simulink model "gm_fft_overlap_tomori"  (R2023b)
settings: Solver=VariableStepAuto  StartTime=0.0  StopTime=inf  RelTol=1e-3
InitFcn:
  | fftparrallelout
  | load('dataram.mat')
  | s= fi(exp(-1j*2*pi.*(0:63)/64),1,16,15);
  | fixed_point = fixdt(1,27,20);
  | fixed_pointu = fixdt(0,29,20);
  | fixed = fixdt(1,22,15);
  | const = fixdt(1,18,17);
  | addConst = fixdt(1,18,16);
  | f =10.4e6;
  | f1=45e6;
  | alpha1 =5;
  | beta1 = 0.00001 ;
  | beta2 = 0.99999 ;
  | beta3 = 23;
undefined symbols (not defined in the file or in its folder): j
libraries: dspxfrm3 x11, commrflib2 x4
(part 1 of 10)
settings Model: Creator=ehsan  LastModifiedBy=mori
settings OptimizationCC: BlockReduction=off  ConditionallyExecuteInputs=off  ReuseModelBlockBuffer=off
settings DebuggingCC: InheritedTsInSrcMsg=none

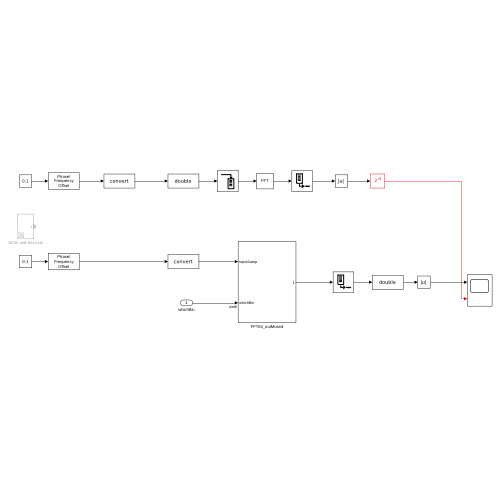
[thumbnail: Simulink's stored preview of the top-level diagram]
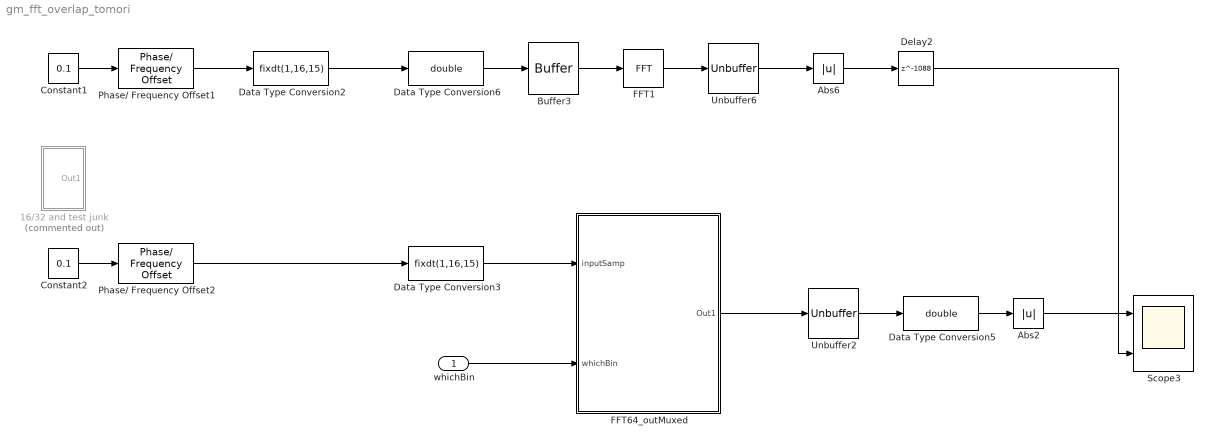
== system gm_fft_overlap_tomori ==
  whichBin : Inport
  16/32 and test junk : Subsystem  Commented=on
  Abs2 : Abs  SaturateOnIntegerOverflow=off
  Abs6 : Abs  SaturateOnIntegerOverflow=off
  Buffer3 : Buffer  V=63  OutputFrames=off
  Constant1 : Constant  Value=0.1  SampleTime=2e-8
  Constant2 : Constant  Value=0.1  SampleTime=2e-8
  Data Type Conversion2 : DataTypeConversion  OutDataTypeStr=fixdt(1,16,15)  SaturateOnIntegerOverflow=off  RndMeth=Floor
  Data Type Conversion3 : DataTypeConversion  OutDataTypeStr=fixdt(1,16,15)  SaturateOnIntegerOverflow=off  RndMeth=Floor
  Data Type Conversion5 : DataTypeConversion  OutDataTypeStr=double  SaturateOnIntegerOverflow=off  RndMeth=Floor
  Data Type Conversion6 : DataTypeConversion  OutDataTypeStr=double  SaturateOnIntegerOverflow=off  RndMeth=Floor
  Delay2 : Delay  DelayLength=1088
  FFT1 : dspxfrm3/FFT  FFTImplementation=Auto  CompMethod=Table lookup  TableOpt=NEW  TableOptActive=Speed  BitRevOrder=off  Normalize=off  InheritFFTLength=on  FFTLength=64  WrapInput=on  roundingMode=Floor  overflowMode=off  firstCoeffDataTypeStr=Inherit: Same word length as input  firstCoeffLastDataTypeStr=Inherit: Same word length as input  outputMin=[]  outputMax=[]
  FFT64_outMuxed : Subsystem
  Phase/ Frequency Offset1 : commrflib2/Phase// Frequency Offset  phaseOffset=0  freqPort=off  freqOffset=1e6
  Phase/ Frequency Offset2 : commrflib2/Phase// Frequency Offset  phaseOffset=0  freqPort=off  freqOffset=1e6
  Scope3 : Scope  NumInputPorts=2
  Unbuffer2 : Unbuffer
  Unbuffer6 : Unbuffer
  wires:
  whichBin/1 -> FFT64_outMuxed/2(whichBin)
  FFT64_outMuxed/1(Out1) -> Unbuffer2/1
  Data Type Conversion3/1 -> FFT64_outMuxed/1(inputSamp)
  Data Type Conversion2/1 -> Data Type Conversion6/1
  Phase/ Frequency Offset1/1 -> Data Type Conversion2/1
  Constant1/1 -> Phase/ Frequency Offset1/1
  Delay2/1 -> Scope3/2
  Abs6/1 -> Delay2/1
  Unbuffer6/1 -> Abs6/1
  FFT1/1 -> Unbuffer6/1
  Buffer3/1 -> FFT1/1
  Abs2/1 -> Scope3/1
  Data Type Conversion5/1 -> Abs2/1
  Unbuffer2/1 -> Data Type Conversion5/1
  Constant2/1 -> Phase/ Frequency Offset2/1
  Phase/ Frequency Offset2/1 -> Data Type Conversion3/1
  Data Type Conversion6/1 -> Buffer3/1

== system gm_fft_overlap_tomori/16//32 and test junk ==
  16 : Subsystem  Commented=on
  16pointfftchan1 : Subsystem  Commented=on
  32 : Subsystem  Commented=on
  Discrete FIR Filter : DiscreteFir  Commented=on  Coefficients=ones(1, 32)
  Real-Imag to Complex : RealImagToComplex  Commented=on
  Sine Wave2 : Sin  Commented=on  Frequency=2*pi*1e6  SampleTime=2e-8
  Sine Wave3 : Sin  Commented=on  Amplitude=.99  Frequency=2*pi*1e6  Phase=pi/2  SampleTime=2e-8
  Out1 : Outport
  wires:
  Real-Imag to Complex/1 -> Out1/1
  Sine Wave3/1 -> Real-Imag to Complex/1
  Sine Wave2/1 -> Real-Imag to Complex/2

== system gm_fft_overlap_tomori/FFT64_outMuxed ==
  inputSamp : Inport
  whichBin : Inport  Port=2  OutDataTypeStr=uint8
  64pointFFTchan : Subsystem
  Multiport Switch1 : MultiPortSwitch  DataPortOrder=Zero-based contiguous  Inputs=64  zeroidx=on  SaturateOnIntegerOverflow=off  InputSameDT=off
  Out1 : Outport
  wires:
  64pointFFTchan/64(Out64) -> Multiport Switch1/65
  64pointFFTchan/63(Out63) -> Multiport Switch1/64
  64pointFFTchan/1(Out1) -> Multiport Switch1/2
  64pointFFTchan/62(Out62) -> Multiport Switch1/63
  64pointFFTchan/2(Out2) -> Multiport Switch1/3
  64pointFFTchan/61(Out61) -> Multiport Switch1/62
  64pointFFTchan/3(Out3) -> Multiport Switch1/4
  64pointFFTchan/60(Out60) -> Multiport Switch1/61
  64pointFFTchan/4(Out4) -> Multiport Switch1/5
  64pointFFTchan/59(Out59) -> Multiport Switch1/60
  64pointFFTchan/5(Out5) -> Multiport Switch1/6
  64pointFFTchan/58(Out58) -> Multiport Switch1/59
  64pointFFTchan/6(Out6) -> Multiport Switch1/7
  64pointFFTchan/57(Out57) -> Multiport Switch1/58
  64pointFFTchan/7(Out7) -> Multiport Switch1/8
  64pointFFTchan/56(Out56) -> Multiport Switch1/57
  64pointFFTchan/8(Out8) -> Multiport Switch1/9
  64pointFFTchan/55(Out55) -> Multiport Switch1/56
  64pointFFTchan/9(Out9) -> Multiport Switch1/10
  64pointFFTchan/54(Out54) -> Multiport Switch1/55
  64pointFFTchan/10(Out10) -> Multiport Switch1/11
  64pointFFTchan/53(Out53) -> Multiport Switch1/54
  64pointFFTchan/11(Out11) -> Multiport Switch1/12
  64pointFFTchan/52(Out52) -> Multiport Switch1/53
  64pointFFTchan/12(Out12) -> Multiport Switch1/13
  64pointFFTchan/51(Out51) -> Multiport Switch1/52
  64pointFFTchan/13(Out13) -> Multiport Switch1/14
  64pointFFTchan/50(Out50) -> Multiport Switch1/51
  64pointFFTchan/14(Out14) -> Multiport Switch1/15
  64pointFFTchan/49(Out49) -> Multiport Switch1/50
  64pointFFTchan/15(Out15) -> Multiport Switch1/16
  64pointFFTchan/48(Out48) -> Multiport Switch1/49
  64pointFFTchan/16(Out16) -> Multiport Switch1/17
  64pointFFTchan/47(Out47) -> Multiport Switch1/48
  64pointFFTchan/17(Out17) -> Multiport Switch1/18
  64pointFFTchan/46(Out46) -> Multiport Switch1/47
  64pointFFTchan/18(Out18) -> Multiport Switch1/19
  64pointFFTchan/45(Out45) -> Multiport Switch1/46
  64pointFFTchan/19(Out19) -> Multiport Switch1/20
  64pointFFTchan/44(Out44) -> Multiport Switch1/45
  64pointFFTchan/20(Out20) -> Multiport Switch1/21
  64pointFFTchan/43(Out43) -> Multiport Switch1/44
  64pointFFTchan/21(Out21) -> Multiport Switch1/22
  64pointFFTchan/42(Out42) -> Multiport Switch1/43
  64pointFFTchan/22(Out22) -> Multiport Switch1/23
  64pointFFTchan/41(Out41) -> Multiport Switch1/42
  64pointFFTchan/23(Out23) -> Multiport Switch1/24
  64pointFFTchan/40(Out40) -> Multiport Switch1/41
  64pointFFTchan/24(Out24) -> Multiport Switch1/25
  64pointFFTchan/39(Out39) -> Multiport Switch1/40
  64pointFFTchan/25(Out25) -> Multiport Switch1/26
  64pointFFTchan/38(Out38) -> Multiport Switch1/39
  64pointFFTchan/26(Out26) -> Multiport Switch1/27
  64pointFFTchan/37(Out37) -> Multiport Switch1/38
  64pointFFTchan/27(Out27) -> Multiport Switch1/28
  64pointFFTchan/36(Out36) -> Multiport Switch1/37
  64pointFFTchan/28(Out28) -> Multiport Switch1/29
  64pointFFTchan/35(Out35) -> Multiport Switch1/36
  64pointFFTchan/29(Out29) -> Multiport Switch1/30
  64pointFFTchan/34(Out34) -> Multiport Switch1/35
  64pointFFTchan/30(Out30) -> Multiport Switch1/31
  64pointFFTchan/33(Out33) -> Multiport Switch1/34
  64pointFFTchan/31(Out31) -> Multiport Switch1/32
  64pointFFTchan/32(Out32) -> Multiport Switch1/33
  whichBin/1 -> Multiport Switch1/1
  inputSamp/1 -> 64pointFFTchan/1(inputSamp)
  Multiport Switch1/1 -> Out1/1

== system gm_fft_overlap_tomori/16//32 and test junk/16 ==
  Abs4 : Abs  SaturateOnIntegerOverflow=off
  Abs5 : Abs  SaturateOnIntegerOverflow=off
  Buffer2 : Buffer  N=16  V=15  OutputFrames=off
  Constant1 : Constant  Value=0.9  SampleTime=2e-8
  Data Type Conversion10 : DataTypeConversion  SaturateOnIntegerOverflow=off  RndMeth=Floor
  Data Type Conversion12 : DataTypeConversion  OutDataTypeStr=double  SaturateOnIntegerOverflow=off  RndMeth=Floor
  Data Type Conversion8 : DataTypeConversion  OutDataTypeStr=fixdt(1,16,15)  SaturateOnIntegerOverflow=off  RndMeth=Floor
  Data Type Conversion9 : DataTypeConversion  OutDataTypeStr=fixdt(1,16,15)  SaturateOnIntegerOverflow=off  RndMeth=Floor
  Delay{34..48} (15 alike) : Delay  DelayLength=1
  Delay49 : Delay  DelayLength=416-272
  FFT16 : Subsystem
  FFT4 : dspxfrm3/FFT  FFTImplementation=Auto  CompMethod=Table lookup  TableOpt=NEW  TableOptActive=Speed  BitRevOrder=off  Normalize=off  InheritFFTLength=on  FFTLength=64  WrapInput=on  roundingMode=Floor  overflowMode=off  firstCoeffDataTypeStr=Inherit: Same word length as input  firstCoeffLastDataTypeStr=Inherit: Same word length as input  outputMin=[]  outputMax=[]
  Mux1 : Mux  Inputs=16
  Phase/ Frequency Offset1 : commrflib2/Phase// Frequency Offset  phaseOffset=pi/2*180/pi  freqPort=off  freqOffset=1e6
  Scope8 : Scope  NumInputPorts=2
  Unbuffer4 : Unbuffer
  Unbuffer5 : Unbuffer
  wires:
  FFT16/14(x13) -> Mux1/14
  Delay37/1 -> Delay38/1, FFT16/5(In5)
  FFT16/12(x11) -> Mux1/12
  Abs4/1 -> Delay49/1
  FFT16/6(x5) -> Mux1/6
  FFT16/16(x15) -> Mux1/16
  FFT16/4(x3) -> Mux1/4
  Buffer2/1 -> FFT4/1
  Delay45/1 -> Delay46/1, FFT16/13(In13)
  FFT16/3(x2) -> Mux1/3
  Delay48/1 -> FFT16/16(In16)
  Delay42/1 -> Delay43/1, FFT16/10(In10)
  Delay36/1 -> Delay37/1, FFT16/4(In4)
  FFT16/1(x0) -> Mux1/1
  FFT16/7(x6) -> Mux1/7
  Delay43/1 -> Delay44/1, FFT16/11(In11)
  FFT16/15(x14) -> Mux1/15
  Data Type Conversion8/1 -> Delay34/1, FFT16/1(In1)
  Delay41/1 -> Delay42/1, FFT16/9(In9)
  Delay34/1 -> Delay35/1, FFT16/2(In2)
  FFT16/9(x8) -> Mux1/9
  FFT16/13(x12) -> Mux1/13
  Delay40/1 -> Delay41/1, FFT16/8(In8)
  Delay49/1 -> Scope8/1
  Unbuffer4/1 -> Abs4/1
  FFT16/2(x1) -> Mux1/2
  FFT16/5(x4) -> Mux1/5
  Data Type Conversion10/1 -> Buffer2/1
  Phase/ Frequency Offset1/1 -> Data Type Conversion8/1, Data Type Conversion9/1
  Mux1/1 -> Unbuffer5/1
  Delay46/1 -> Delay47/1, FFT16/14(In14)
  Delay39/1 -> Delay40/1, FFT16/7(In7)
  Data Type Conversion9/1 -> Data Type Conversion10/1
  Delay47/1 -> Delay48/1, FFT16/15(In15)
  Constant1/1 -> Phase/ Frequency Offset1/1
  FFT16/8(x7) -> Mux1/8
  FFT16/10(x9) -> Mux1/10
  FFT16/11(x10) -> Mux1/11
  Unbuffer5/1 -> Data Type Conversion12/1
  Delay44/1 -> Delay45/1, FFT16/12(In12)
  Data Type Conversion12/1 -> Abs5/1
  Delay35/1 -> Delay36/1, FFT16/3(In3)
  Delay38/1 -> Delay39/1, FFT16/6(In6)
  Abs5/1 -> Scope8/2
  FFT4/1 -> Unbuffer4/1

== system gm_fft_overlap_tomori/16//32 and test junk/16pointfftchan1 ==
  Input : Inport
      settings: SignalType=complex
  Delay{10..24} (15 alike) : Delay  DelayLength=1
  fft_res : Subsystem
  Out1 : Outport
  wires:
  Delay24/1 -> fft_res/16(In16)
  Delay11/1 -> Delay12/1, fft_res/3(In3)
  Delay15/1 -> fft_res/7(In7), Delay16/1
  Delay13/1 -> fft_res/5(In5), Delay14/1
  Delay20/1 -> fft_res/12(In12), Delay21/1
  Delay14/1 -> fft_res/6(In6), Delay15/1
  Delay22/1 -> fft_res/14(In14), Delay23/1
  Delay19/1 -> fft_res/11(In11), Delay20/1
  Delay23/1 -> fft_res/15(In15), Delay24/1
  Input/1 -> fft_res/1(In1), Delay10/1
  Delay12/1 -> fft_res/4(In4), Delay13/1
  Delay17/1 -> Delay18/1, fft_res/9(In9)
  Delay10/1 -> Delay11/1, fft_res/2(In2)
  Delay18/1 -> fft_res/10(In10), Delay19/1
  fft_res/1(Out1) -> Out1/1
  Delay16/1 -> fft_res/8(In8), Delay17/1
  Delay21/1 -> fft_res/13(In13), Delay22/1

== system gm_fft_overlap_tomori/16//32 and test junk/32 ==
  In1 : Inport
  Abs1 : Abs  SaturateOnIntegerOverflow=off
  Abs3 : Abs  SaturateOnIntegerOverflow=off
  Buffer : Buffer  Commented=on  V=63  OutputFrames=off
  Buffer1 : Buffer  N=32  V=31  OutputFrames=off
  Constant : Constant  Value=0.1  SampleTime=2e-8
  Data Type Conversion : DataTypeConversion  Commented=on  OutDataTypeStr=fixdt(1,16,15)  SaturateOnIntegerOverflow=off  RndMeth=Floor
  Data Type Conversion1 : DataTypeConversion  OutDataTypeStr=fixdt(1,16,15)  SaturateOnIntegerOverflow=off  RndMeth=Floor
  Data Type Conversion4 : DataTypeConversion  OutDataTypeStr=double  SaturateOnIntegerOverflow=off  RndMeth=Floor
  Delay1 : Delay  DelayLength=416
  Delay{3..33} (31 alike) : Delay  DelayLength=1
  FFT : dspxfrm3/FFT  Commented=on  FFTImplementation=Auto  CompMethod=Table lookup  TableOpt=NEW  TableOptActive=Speed  BitRevOrder=off  Normalize=off  InheritFFTLength=on  FFTLength=64  WrapInput=on  roundingMode=Floor  overflowMode=off  firstCoeffDataTypeStr=Inherit: Same word length as input  firstCoeffLastDataTypeStr=Inherit: Same word length as input  outputMin=[]  outputMax=[]
  FFT2 : dspxfrm3/FFT  FFTImplementation=Auto  CompMethod=Table lookup  TableOpt=NEW  TableOptActive=Speed  BitRevOrder=off  Normalize=off  InheritFFTLength=on  FFTLength=64  WrapInput=on  roundingMode=Floor  overflowMode=off  firstCoeffDataTypeStr=Inherit: Same word length as input  firstCoeffLastDataTypeStr=Inherit: Same word length as input  outputMin=[]  outputMax=[]
  FFT32 : Subsystem
  Mux : Mux  Inputs=32
  Phase/ Frequency Offset : commrflib2/Phase// Frequency Offset  phaseOffset=0  freqPort=off  freqOffset=1e6
  Scope : Scope  Commented=on
  Scope1 : Scope  NumInputPorts=2
  Scope10 : Scope  NumInputPorts=2
  Scope2 : Scope
  Sine Wave : Sin  Commented=on  Frequency=2*pi*12.5e6  SampleTime=0
  Spectrum Analyzer : SpectrumAnalyzer  Commented=on
  Unbuffer1 : Unbuffer
  Unbuffer3 : Unbuffer
  wires:
  FFT32/6(x5) -> Mux/6
  In1/1 -> Buffer1/1
  FFT32/17(x16) -> Mux/17
  Buffer/1 -> FFT/1
  FFT32/9(x8) -> Mux/9
  Delay25/1 -> FFT32/25(In25), Delay26/1
  Delay14/1 -> Delay15/1, FFT32/6(In6)
  Delay26/1 -> FFT32/26(In26), Delay27/1
  FFT32/21(x20) -> Mux/21
  Data Type Conversion4/1 -> Scope10/2, Abs1/1
  Delay13/1 -> Delay14/1, FFT32/5(In5)
  FFT32/31(x30) -> Mux/31
  Delay22/1 -> Delay23/1, FFT32/14(In14)
  Delay9/1 -> FFT32/24(In24), Delay25/1
  FFT32/2(x1) -> Mux/2
  Unbuffer3/1 -> Scope10/1, Abs3/1
  FFT/1 -> Spectrum Analyzer/1
  FFT32/28(x27) -> Mux/28
  Data Type Conversion/1 -> Scope/1, Buffer/1
  FFT32/1(x0) -> Mux/1
  Delay3/1 -> FFT32/17(In19), Delay33/1
  Delay24/1 -> Delay3/1, FFT32/16(In17)
  Delay32/1 -> FFT32/32(In32)
  Delay18/1 -> Delay19/1, FFT32/10(In10)
  Phase/ Frequency Offset/1 -> Data Type Conversion1/1
  FFT32/18(x17) -> Mux/18
  Delay29/1 -> FFT32/29(In29), Delay30/1
  Abs1/1 -> Scope2/1, Scope1/1
  Delay6/1 -> FFT32/21(In21), Delay7/1
  Mux/1 -> Unbuffer1/1
  FFT32/23(x22) -> Mux/23
  Delay30/1 -> FFT32/30(In30), Delay31/1
  FFT32/20(x19) -> Mux/20
  Delay1/1 -> Scope1/2
  Delay5/1 -> FFT32/20(In20), Delay6/1
  Delay17/1 -> Delay18/1, FFT32/9(In9)
  Delay27/1 -> FFT32/27(In27), Delay28/1
  FFT32/8(x7) -> Mux/8
  Sine Wave/1 -> Data Type Conversion/1
  Delay23/1 -> Delay24/1, FFT32/15(In15)
  Delay20/1 -> Delay21/1, FFT32/12(In12)
  FFT32/10(x9) -> Mux/10
  Delay12/1 -> Delay13/1, FFT32/4(In4)
  Unbuffer1/1 -> Data Type Conversion4/1
  FFT32/29(x28) -> Mux/29
  Delay33/1 -> FFT32/18(In16), Delay4/1
  Delay19/1 -> Delay20/1, FFT32/11(In11)
  FFT32/27(x26) -> Mux/27
  FFT32/25(x24) -> Mux/25
  Data Type Conversion1/1 -> Delay10/1, FFT32/1(In1)
  Delay4/1 -> FFT32/19(In18), Delay5/1
  FFT32/30(x29) -> Mux/30
  Constant/1 -> Phase/ Frequency Offset/1
  Delay15/1 -> Delay16/1, FFT32/7(In7)
  Delay11/1 -> Delay12/1, FFT32/3(In3)
  FFT2/1 -> Unbuffer3/1
  FFT32/19(x18) -> Mux/19
  FFT32/11(x10) -> Mux/11
  FFT32/13(x12) -> Mux/13
  Delay8/1 -> FFT32/23(In23), Delay9/1
  Delay7/1 -> FFT32/22(In22), Delay8/1
  Delay10/1 -> Delay11/1, FFT32/2(In2)
  Delay31/1 -> FFT32/31(In31), Delay32/1
  Delay16/1 -> Delay17/1, FFT32/8(In8)
  FFT32/3(x2) -> Mux/3
  FFT32/24(x23) -> Mux/24
  Delay28/1 -> FFT32/28(In28), Delay29/1
  FFT32/5(x4) -> Mux/5
  FFT32/14(x13) -> Mux/14
  Delay21/1 -> Delay22/1, FFT32/13(In13)
  FFT32/32(x31) -> Mux/32
  FFT32/15(x14) -> Mux/15
  FFT32/12(x11) -> Mux/12
  FFT32/4(x3) -> Mux/4
  FFT32/16(x15) -> Mux/16
  Buffer1/1 -> FFT2/1
  FFT32/22(x21) -> Mux/22
  Abs3/1 -> Delay1/1
  FFT32/26(x25) -> Mux/26
  FFT32/7(x6) -> Mux/7

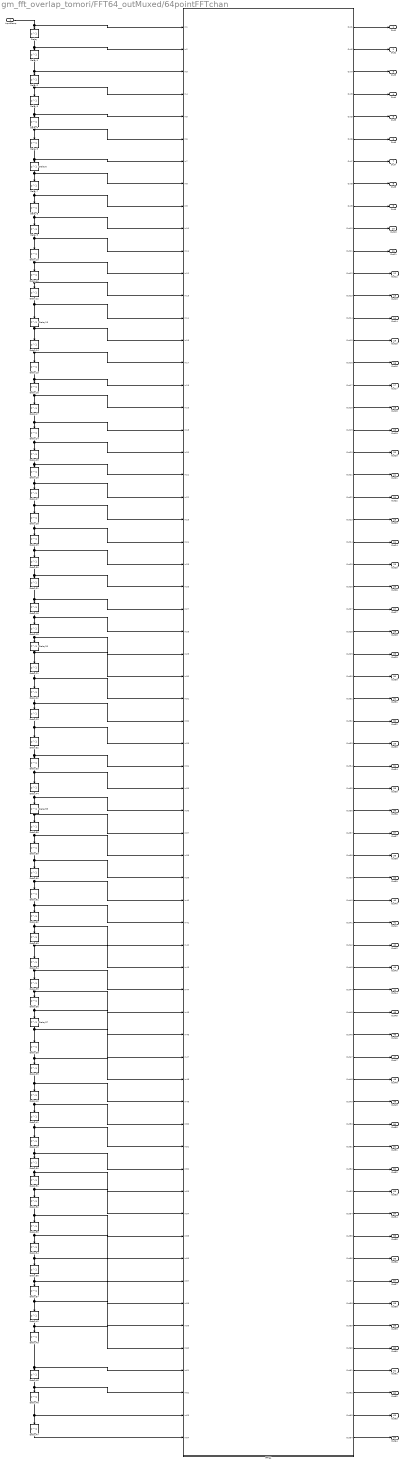
== system gm_fft_overlap_tomori/FFT64_outMuxed/64pointFFTchan ==
  inputSamp : Inport  OutDataTypeStr=fixdt(1,16, 15)
  Delay{,1..47,49..63} (63 alike) : Delay  DelayLength=1
  FFT64 : Subsystem
  Out1 : Outport  VectorParamsAs1DForOutWhenUnconnected=off
  Out2 : Outport  Port=2  VectorParamsAs1DForOutWhenUnconnected=off
  Out3 : Outport  Port=3  VectorParamsAs1DForOutWhenUnconnected=off
  Out4 : Outport  Port=4  VectorParamsAs1DForOutWhenUnconnected=off
  Out5 : Outport  Port=5  VectorParamsAs1DForOutWhenUnconnected=off
  Out6 : Outport  Port=6  VectorParamsAs1DForOutWhenUnconnected=off
  Out7 : Outport  Port=7  VectorParamsAs1DForOutWhenUnconnected=off
  Out8 : Outport  Port=8  VectorParamsAs1DForOutWhenUnconnected=off
  Out9 : Outport  Port=9  VectorParamsAs1DForOutWhenUnconnected=off
  Out10 : Outport  Port=10  VectorParamsAs1DForOutWhenUnconnected=off
  Out11 : Outport  Port=11  VectorParamsAs1DForOutWhenUnconnected=off
  Out12 : Outport  Port=12  VectorParamsAs1DForOutWhenUnconnected=off
  Out13 : Outport  Port=13  VectorParamsAs1DForOutWhenUnconnected=off
  Out14 : Outport  Port=14  VectorParamsAs1DForOutWhenUnconnected=off
  Out15 : Outport  Port=15  VectorParamsAs1DForOutWhenUnconnected=off
  Out16 : Outport  Port=16  VectorParamsAs1DForOutWhenUnconnected=off
  Out17 : Outport  Port=17  VectorParamsAs1DForOutWhenUnconnected=off
  Out18 : Outport  Port=18  VectorParamsAs1DForOutWhenUnconnected=off
  Out19 : Outport  Port=19  VectorParamsAs1DForOutWhenUnconnected=off
  Out20 : Outport  Port=20  VectorParamsAs1DForOutWhenUnconnected=off
  Out21 : Outport  Port=21  VectorParamsAs1DForOutWhenUnconnected=off
  Out22 : Outport  Port=22  VectorParamsAs1DForOutWhenUnconnected=off
  Out23 : Outport  Port=23  VectorParamsAs1DForOutWhenUnconnected=off
  Out24 : Outport  Port=24  VectorParamsAs1DForOutWhenUnconnected=off
  Out25 : Outport  Port=25  VectorParamsAs1DForOutWhenUnconnected=off
  Out26 : Outport  Port=26  VectorParamsAs1DForOutWhenUnconnected=off
  Out27 : Outport  Port=27  VectorParamsAs1DForOutWhenUnconnected=off
  Out28 : Outport  Port=28  VectorParamsAs1DForOutWhenUnconnected=off
  Out29 : Outport  Port=29  VectorParamsAs1DForOutWhenUnconnected=off
  Out30 : Outport  Port=30  VectorParamsAs1DForOutWhenUnconnected=off
  Out31 : Outport  Port=31  VectorParamsAs1DForOutWhenUnconnected=off
  Out32 : Outport  Port=32  VectorParamsAs1DForOutWhenUnconnected=off
  Out33 : Outport  Port=33  VectorParamsAs1DForOutWhenUnconnected=off
  Out34 : Outport  Port=34  VectorParamsAs1DForOutWhenUnconnected=off
  Out35 : Outport  Port=35  VectorParamsAs1DForOutWhenUnconnected=off
  Out36 : Outport  Port=36  VectorParamsAs1DForOutWhenUnconnected=off
  Out37 : Outport  Port=37  VectorParamsAs1DForOutWhenUnconnected=off
  Out38 : Outport  Port=38  VectorParamsAs1DForOutWhenUnconnected=off
  Out39 : Outport  Port=39  VectorParamsAs1DForOutWhenUnconnected=off
  Out40 : Outport  Port=40  VectorParamsAs1DForOutWhenUnconnected=off
  Out41 : Outport  Port=41  VectorParamsAs1DForOutWhenUnconnected=off
  Out42 : Outport  Port=42  VectorParamsAs1DForOutWhenUnconnected=off
  Out43 : Outport  Port=43  VectorParamsAs1DForOutWhenUnconnected=off
  Out44 : Outport  Port=44  VectorParamsAs1DForOutWhenUnconnected=off
  Out45 : Outport  Port=45  VectorParamsAs1DForOutWhenUnconnected=off
  Out46 : Outport  Port=46  VectorParamsAs1DForOutWhenUnconnected=off
  Out47 : Outport  Port=47  VectorParamsAs1DForOutWhenUnconnected=off
  Out48 : Outport  Port=48  VectorParamsAs1DForOutWhenUnconnected=off
  Out49 : Outport  Port=49  VectorParamsAs1DForOutWhenUnconnected=off
  Out50 : Outport  Port=50  VectorParamsAs1DForOutWhenUnconnected=off
  Out51 : Outport  Port=51  VectorParamsAs1DForOutWhenUnconnected=off
  Out52 : Outport  Port=52  VectorParamsAs1DForOutWhenUnconnected=off
  Out53 : Outport  Port=53  VectorParamsAs1DForOutWhenUnconnected=off
  Out54 : Outport  Port=54  VectorParamsAs1DForOutWhenUnconnected=off
  Out55 : Outport  Port=55  VectorParamsAs1DForOutWhenUnconnected=off
  Out56 : Outport  Port=56  VectorParamsAs1DForOutWhenUnconnected=off
  Out57 : Outport  Port=57  VectorParamsAs1DForOutWhenUnconnected=off
  Out58 : Outport  Port=58  VectorParamsAs1DForOutWhenUnconnected=off
  Out59 : Outport  Port=59  VectorParamsAs1DForOutWhenUnconnected=off
  Out60 : Outport  Port=60  VectorParamsAs1DForOutWhenUnconnected=off
  Out61 : Outport  Port=61  VectorParamsAs1DForOutWhenUnconnected=off
  Out62 : Outport  Port=62  VectorParamsAs1DForOutWhenUnconnected=off
  Out63 : Outport  Port=63  VectorParamsAs1DForOutWhenUnconnected=off
  Out64 : Outport  Port=64  VectorParamsAs1DForOutWhenUnconnected=off
  wires:
  FFT64/64(Out64) -> Out64/1
  FFT64/63(Out63) -> Out63/1
  FFT64/62(Out62) -> Out62/1
  FFT64/61(Out61) -> Out61/1
  FFT64/60(Out60) -> Out60/1
  FFT64/59(Out59) -> Out59/1
  FFT64/58(Out58) -> Out58/1
  FFT64/57(Out57) -> Out57/1
  FFT64/56(Out56) -> Out56/1
  FFT64/55(Out55) -> Out55/1
  FFT64/54(Out54) -> Out54/1
  FFT64/53(Out53) -> Out53/1
  FFT64/52(Out52) -> Out52/1
  FFT64/51(Out51) -> Out51/1
  FFT64/50(Out50) -> Out50/1
  FFT64/49(Out49) -> Out49/1
  FFT64/48(Out48) -> Out48/1
  FFT64/47(Out47) -> Out47/1
  FFT64/46(Out46) -> Out46/1
  FFT64/45(Out45) -> Out45/1
  FFT64/44(Out44) -> Out44/1
  FFT64/43(Out43) -> Out43/1
  FFT64/42(Out42) -> Out42/1
  FFT64/41(Out41) -> Out41/1
  FFT64/40(Out40) -> Out40/1
  FFT64/39(Out39) -> Out39/1
  FFT64/38(Out38) -> Out38/1
  FFT64/37(Out37) -> Out37/1
  FFT64/36(Out36) -> Out36/1
  FFT64/35(Out35) -> Out35/1
  FFT64/34(Out34) -> Out34/1
  FFT64/33(Out33) -> Out33/1
  FFT64/32(Out32) -> Out32/1
  FFT64/31(Out31) -> Out31/1
  FFT64/30(Out30) -> Out30/1
  FFT64/29(Out29) -> Out29/1
  FFT64/28(Out28) -> Out28/1
  FFT64/27(Out27) -> Out27/1
  FFT64/26(Out26) -> Out26/1
  FFT64/25(Out25) -> Out25/1
  FFT64/24(Out24) -> Out24/1
  FFT64/23(Out23) -> Out23/1
  FFT64/22(Out22) -> Out22/1
  FFT64/21(Out21) -> Out21/1
  FFT64/20(Out20) -> Out20/1
  FFT64/19(Out19) -> Out19/1
  FFT64/18(Out18) -> Out18/1
  FFT64/17(Out17) -> Out17/1
  FFT64/16(Out16) -> Out16/1
  FFT64/15(Out15) -> Out15/1
  FFT64/14(Out14) -> Out14/1
  FFT64/13(Out13) -> Out13/1
  FFT64/12(Out12) -> Out12/1
  FFT64/11(Out11) -> Out11/1
  FFT64/10(Out10) -> Out10/1
  FFT64/9(Out9) -> Out9/1
  FFT64/8(Out8) -> Out8/1
  FFT64/7(Out7) -> Out7/1
  FFT64/6(Out6) -> Out6/1
  FFT64/5(Out5) -> Out5/1
  FFT64/4(Out3) -> Out4/1
  FFT64/3(Out4) -> Out3/1
  FFT64/2(Out2) -> Out2/1
  FFT64/1(Out1) -> Out1/1
  Delay47/1 -> FFT64/64(In64)
  Delay23/1 -> Delay32/1, FFT64/33(In33)
  Delay32/1 -> Delay33/1, FFT64/34(In34)
  Delay44/1 -> Delay55/1, FFT64/36(In36)
  Delay33/1 -> Delay44/1, FFT64/35(In35)
  Delay58/1 -> Delay59/1, FFT64/38(In38)
  Delay59/1 -> Delay60/1, FFT64/39(In39)
  Delay60/1 -> Delay61/1, FFT64/40(In40)
  Delay55/1 -> Delay58/1, FFT64/37(In37)
  Delay35/1 -> Delay36/1, FFT64/45(In45)
  Delay38/1 -> Delay39/1, FFT64/48(In48)
  Delay37/1 -> Delay38/1, FFT64/47(In47)
  Delay36/1 -> Delay37/1, FFT64/46(In46)
  Delay63/1 -> Delay34/1, FFT64/43(In43)
  Delay34/1 -> Delay35/1, FFT64/44(In44)
  Delay62/1 -> Delay63/1, FFT64/42(In42)
  Delay61/1 -> Delay62/1, FFT64/41(In41)
  Delay42/1 -> Delay43/1, FFT64/60(In60)
  Delay56/1 -> Delay57/1, FFT64/58(In58)
  Delay45/1 -> Delay46/1, FFT64/62(In62)
  Delay50/1 -> Delay51/1, FFT64/53(In53)
  Delay49/1 -> Delay50/1, FFT64/52(In52)
  Delay51/1 -> Delay52/1, FFT64/54(In54)
  Delay41/1 -> Delay49/1, FFT64/51(In51)
  Delay46/1 -> Delay47/1, FFT64/63(In63)
  Delay53/1 -> Delay54/1, FFT64/56(In56)
  Delay57/1 -> Delay42/1, FFT64/59(In59)
  Delay52/1 -> Delay53/1, FFT64/55(In55)
  Delay43/1 -> Delay45/1, FFT64/61(In61)
  Delay40/1 -> Delay41/1, FFT64/50(In50)
  Delay54/1 -> Delay56/1, FFT64/57(In57)
  Delay39/1 -> Delay40/1, FFT64/49(In49)
  Delay15/1 -> Delay16/1, FFT64/17(In19)
  Delay29/1 -> Delay30/1, FFT64/25(In25)
  Delay16/1 -> Delay17/1, FFT64/18(In16)
  Delay19/1 -> Delay20/1, FFT64/29(In29)
  Delay27/1 -> Delay28/1, FFT64/23(In23)
  Delay31/1 -> Delay18/1, FFT64/27(In27)
  Delay28/1 -> Delay29/1, FFT64/24(In24)
  Delay21/1 -> Delay22/1, FFT64/31(In31)
  Delay17/1 -> Delay24/1, FFT64/19(In18)
  Delay26/1 -> Delay27/1, FFT64/22(In22)
  Delay24/1 -> Delay25/1, FFT64/20(In20)
  Delay22/1 -> Delay23/1, FFT64/32(In32)
  Delay25/1 -> Delay26/1, FFT64/21(In21)
  Delay20/1 -> Delay21/1, FFT64/30(In30)
  Delay30/1 -> Delay31/1, FFT64/26(In26)
  Delay18/1 -> Delay19/1, FFT64/28(In28)
  Delay7/1 -> Delay8/1, FFT64/9(In9)
  Delay8/1 -> Delay9/1, FFT64/10(In10)
  Delay10/1 -> Delay11/1, FFT64/12(In12)
  Delay9/1 -> Delay10/1, FFT64/11(In11)
  Delay12/1 -> Delay13/1, FFT64/14(In14)
  Delay13/1 -> Delay14/1, FFT64/15(In15)
  Delay14/1 -> Delay15/1, FFT64/16(In17)
  Delay11/1 -> Delay12/1, FFT64/13(In13)
  Delay3/1 -> Delay4/1, FFT64/5(In5)
  Delay6/1 -> Delay7/1, FFT64/8(In8)
  Delay5/1 -> Delay6/1, FFT64/7(In7)
  Delay4/1 -> Delay5/1, FFT64/6(In6)
  Delay1/1 -> Delay2/1, FFT64/3(In3)
  Delay2/1 -> Delay3/1, FFT64/4(In4)
  Delay/1 -> Delay1/1, FFT64/2(In2)
  inputSamp/1 -> Delay/1, FFT64/1(In1)

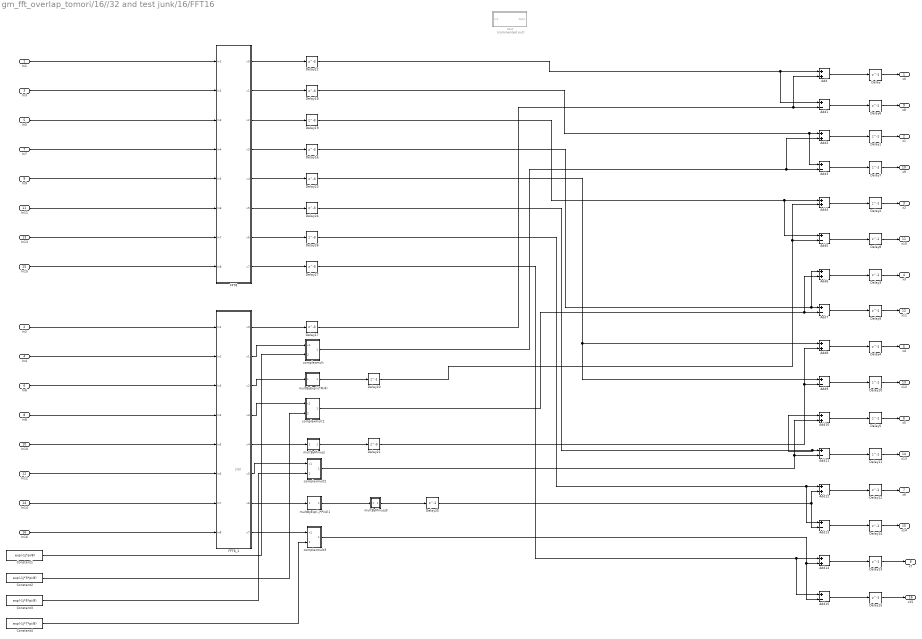
== system gm_fft_overlap_tomori/16//32 and test junk/16/FFT16 ==
  note: s(5)
  In1 : Inport
  In2 : Inport  Port=2
  In3 : Inport  Port=3
  In4 : Inport  Port=4
  In5 : Inport  Port=5
  In6 : Inport  Port=6
  In7 : Inport  Port=7
  In8 : Inport  Port=8
  In9 : Inport  Port=9
  In10 : Inport  Port=10
  In11 : Inport  Port=11
  In12 : Inport  Port=12
  In13 : Inport  Port=13
  In14 : Inport  Port=14
  In15 : Inport  Port=15
  In16 : Inport  Port=16
  Add{,2,4,6,8,10,12,14} (8 alike) : Sum  OutDataTypeStr=fixed
  Add{1,3,5,7,9,11,13,15} (8 alike) : Sum  Inputs=+-  OutDataTypeStr=fixed
  Constant1 : Constant  Value=exp(-1j*pi/8)  OutDataTypeStr=fixed  SampleTime=-1
  Constant2 : Constant  Value=exp(-1j*3*pi/8)  OutDataTypeStr=fixed  SampleTime=-1
  Constant3 : Constant  Value=exp(-1j*5*pi/8)  OutDataTypeStr=fixed  SampleTime=-1
  Constant4 : Constant  Value=exp(-1j*7*pi/8)  OutDataTypeStr=fixed  SampleTime=-1
  Delay{,1..15,20,25} (18 alike) : Delay  DelayLength=1
  Delay{16..19,21..24,26..27} (10 alike) : Delay  DelayLength=3
  FFT8 : Subsystem
  FFT8_1 : Subsystem
  complexmult : Subsystem
  complexmult1 : Subsystem
  complexmult2 : Subsystem
  complexmult3 : Subsystem
  multByExp(-j*Pi/4) : Subsystem
  multByExp(-j*Pi/4)1 : Subsystem
  multByMinusJ : Subsystem
  multByMinusJ3 : Subsystem
  test : Subsystem  Commented=on
  x0 : Outport
  x1 : Outport  Port=2
  x2 : Outport  Port=3
  x3 : Outport  Port=4
  x4 : Outport  Port=5
  x5 : Outport  Port=6
  x6 : Outport  Port=7
  x7 : Outport  Port=8
  x8 : Outport  Port=9
  x9 : Outport  Port=10
  x10 : Outport  Port=11
  x11 : Outport  Port=12
  x12 : Outport  Port=13
  x13 : Outport  Port=14
  x14 : Outport  Port=15
  x15 : Outport  Port=16
  wires:
  In16/1 -> FFT8_1/8(In8)
  In14/1 -> FFT8_1/7(In7)
  In12/1 -> FFT8_1/6(In6)
  In10/1 -> FFT8_1/5(In5)
  In8/1 -> FFT8_1/4(In4)
  In6/1 -> FFT8_1/3(In3)
  In4/1 -> FFT8_1/2(In2)
  In2/1 -> FFT8_1/1(In1)
  In15/1 -> FFT8/8(In8)
  In13/1 -> FFT8/7(In7)
  In11/1 -> FFT8/6(In6)
  In9/1 -> FFT8/5(In5)
  In7/1 -> FFT8/4(In4)
  In5/1 -> FFT8/3(In3)
  In3/1 -> FFT8/2(In2)
  In1/1 -> FFT8/1(In1)
  multByExp(-j*Pi/4)1/1(Out1) -> multByMinusJ3/1(In1)
  Constant3/1 -> complexmult2/2(In3)
  FFT8_1/6(x5) -> complexmult2/1(x1)
  Delay27/1 -> Add14/1, Add15/1
  Delay26/1 -> Add12/1, Add13/1
  Add15/1 -> Delay15/1
  Add14/1 -> Delay13/1
  FFT8/8(x7) -> Delay27/1
  complexmult3/1(Out1) -> Add14/2, Add15/2
  FFT8_1/8(x7) -> complexmult3/1(x1)
  Constant4/1 -> complexmult3/2(In3)
  Add13/1 -> Delay14/1
  Add12/1 -> Delay12/1
  Delay25/1 -> Add13/2, Add12/2
  FFT8/7(x6) -> Delay26/1
  multByMinusJ3/1(Out1) -> Delay25/1
  FFT8_1/7(x6) -> multByExp(-j*Pi/4)1/1(In1)
  Delay24/1 -> Add11/1, Add10/1
  Delay23/1 -> Add8/1, Add9/1
  Delay16/1 -> Add7/1, Add6/1
  Delay22/1 -> Add/1, Add1/1
  FFT8_1/5(x4) -> multByMinusJ/1(x4)
  Delay21/1 -> Add8/2, Add9/2
  Delay19/1 -> Add4/1, Add5/1
  Delay20/1 -> Add5/2, Add4/2
  Delay18/1 -> Add2/1, Add3/1
  Delay17/1 -> Add1/2, Add/2
  FFT8/1(x0) -> Delay22/1
  Delay15/1 -> x15/1
  Delay14/1 -> x14/1
  Delay13/1 -> x7/1
  Delay12/1 -> x6/1
  Delay11/1 -> x13/1
  Delay10/1 -> x12/1
  Delay9/1 -> x11/1
  Delay8/1 -> x10/1
  Delay7/1 -> x9/1
  Delay6/1 -> x8/1
  Delay5/1 -> x5/1
  Delay4/1 -> x4/1
  Delay3/1 -> x3/1
  Delay2/1 -> x2/1
  Delay1/1 -> x1/1
  Delay/1 -> x0/1
  Add11/1 -> Delay11/1
  Add10/1 -> Delay5/1
  FFT8/6(x5) -> Delay24/1
  complexmult2/1(Out1) -> Add10/2, Add11/2
  Add9/1 -> Delay10/1
  Add8/1 -> Delay4/1
  multByMinusJ/1(Out1) -> Delay21/1
  FFT8/5(x4) -> Delay23/1
  Add7/1 -> Delay9/1
  Add6/1 -> Delay3/1
  complexmult1/1(Out1) -> Add7/2, Add6/2
  FFT8/4(x3) -> Delay16/1
  FFT8_1/4(x3) -> complexmult1/1(x1)
  Constant2/1 -> complexmult1/2(In3)
  multByExp(-j*Pi/4)/1(Out1) -> Delay20/1
  Add5/1 -> Delay8/1
  Add4/1 -> Delay2/1
  FFT8/3(x2) -> Delay19/1
  FFT8_1/3(x2) -> multByExp(-j*Pi/4)/1(In1)
  Add3/1 -> Delay7/1
  complexmult/1(Out1) -> Add3/2, Add2/2
  Add2/1 -> Delay1/1
  FFT8/2(x1) -> Delay18/1
  FFT8_1/2(x1) -> complexmult/1(x1)
  Constant1/1 -> complexmult/2(In3)
  Add1/1 -> Delay6/1
  Add/1 -> Delay/1
  FFT8_1/1(x0) -> Delay17/1

== system gm_fft_overlap_tomori/16//32 and test junk/16pointfftchan1/fft_res ==
  In1 : Inport
  In2 : Inport  Port=2
  In3 : Inport  Port=3
  In4 : Inport  Port=4
  In5 : Inport  Port=5
  In6 : Inport  Port=6
  In7 : Inport  Port=7
  In8 : Inport  Port=8
  In9 : Inport  Port=9
  In10 : Inport  Port=10
  In11 : Inport  Port=11
  In12 : Inport  Port=12
  In13 : Inport  Port=13
  In14 : Inport  Port=14
  In15 : Inport  Port=15
  In16 : Inport  Port=16
  Add{1..7,16} (8 alike) : Sum  OutDataTypeStr=fixed_point  AccumDataTypeStr=fixed_point
  Add{8..14,21} (8 alike) : Sum  Inputs=+-  OutDataTypeStr=fixed_point  AccumDataTypeStr=fixed_point
  Delay{1..9,12} (10 alike) : Delay  DelayLength=3
  Delay{10..11,13..26} (16 alike) : Delay  DelayLength=1
  Demux : Demux  Outputs=8
  Demux1 : Demux  Outputs=8
  Mux : Mux  Inputs=16
  cmut1 : Subsystem
  cmut2 : Subsystem
  cmut21 : Subsystem
  cmut3 : Subsystem
  fft_1 : Subsystem
  fft_8 : Subsystem
  prod_2 : Subsystem
  prod_3 : Subsystem
  s2 : Subsystem
  Out1 : Outport
  wires:
  Delay26/1 -> cmut3/1(In1)
  Delay25/1 -> prod_3/1(In1)
  Delay24/1 -> cmut2/1(In1)
  Delay23/1 -> s2/1(In1)
  Delay22/1 -> cmut1/1(In1)
  Delay21/1 -> prod_2/1(In1)
  Delay20/1 -> cmut21/1(In1)
  Delay19/1 -> Delay8/1
  Delay18/1 -> Delay7/1
  Delay17/1 -> Delay6/1
  Delay16/1 -> Delay5/1
  Delay15/1 -> Delay4/1
  Delay14/1 -> Delay3/1
  Delay13/1 -> Delay2/1
  Delay11/1 -> Delay1/1
  Delay10/1 -> Delay12/1
  fft_8/1(Out1) -> Demux/1
  prod_3/1(Out1) -> fft_1/7(In7)
  Demux/8 -> Mux/8
  fft_1/1(Out1) -> Demux1/1
  Demux1/6 -> Mux/14
  Demux/4 -> Mux/4
  In10/1 -> Add8/2, Add1/2
  In4/1 -> Add10/1, Add3/1
  Demux1/7 -> Mux/15
  Demux/3 -> Mux/3
  prod_2/1(Out1) -> fft_1/3(In3)
  In6/1 -> Add12/1, Add5/1
  Demux1/2 -> Mux/10
  Demux1/4 -> Mux/12
  In12/1 -> Add10/2, Add3/2
  In8/1 -> Add14/1, Add7/1
  In1/1 -> Add21/1, Add16/1
  Demux1/8 -> Mux/16
  In13/1 -> Add11/2, Add4/2
  In9/1 -> Add21/2, Add16/2
  Mux/1 -> Out1/1
  In5/1 -> Add11/1, Add4/1
  In3/1 -> Add9/1, Add2/1
  In11/1 -> Add9/2, Add2/2
  Demux1/5 -> Mux/13
  In16/1 -> Add14/2, Add7/2
  In2/1 -> Add8/1, Add1/1
  s2/1(Out1) -> Delay9/1
  In7/1 -> Add13/1, Add6/1
  Demux/1 -> Mux/1
  Demux/6 -> Mux/6
  Demux/5 -> Mux/5
  In15/1 -> Add13/2, Add6/2
  In14/1 -> Add12/2, Add5/2
  Demux1/1 -> Mux/9
  Demux/2 -> Mux/2
  Demux1/3 -> Mux/11
  Demux/7 -> Mux/7
  Delay12/1 -> fft_8/1(In1)
  Delay1/1 -> fft_8/2(In2)
  Delay2/1 -> fft_8/3(In3)
  Delay3/1 -> fft_8/4(In4)
  Delay4/1 -> fft_8/5(In5)
  Delay5/1 -> fft_8/6(In6)
  Delay6/1 -> fft_8/7(In7)
  Delay7/1 -> fft_8/8(In8)
  Delay8/1 -> fft_1/1(In1)
  Delay9/1 -> fft_1/5(In5)
  cmut21/1(Out1) -> fft_1/2(In2)
  Add16/1 -> Delay10/1
  Add1/1 -> Delay11/1
  Add2/1 -> Delay13/1
  Add3/1 -> Delay14/1
  Add4/1 -> Delay15/1
  Add5/1 -> Delay16/1
  Add6/1 -> Delay17/1
  Add7/1 -> Delay18/1
  Add21/1 -> Delay19/1
  Add8/1 -> Delay20/1
  Add9/1 -> Delay21/1
  Add11/1 -> Delay23/1
  Add13/1 -> Delay25/1
  Add10/1 -> Delay22/1
  cmut1/1(Out1) -> fft_1/4(In4)
  Add12/1 -> Delay24/1
  cmut2/1(Out1) -> fft_1/6(In6)
  Add14/1 -> Delay26/1
  cmut3/1(Out1) -> fft_1/8(In8)

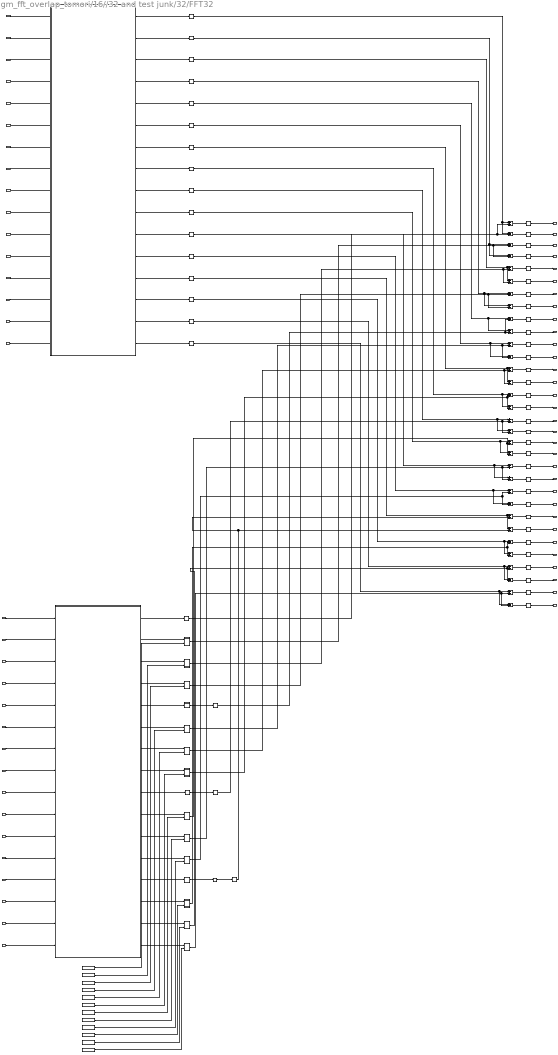
== system gm_fft_overlap_tomori/16//32 and test junk/32/FFT32 ==
  In1 : Inport
  In2 : Inport  Port=2
  In3 : Inport  Port=3
  In4 : Inport  Port=4
  In5 : Inport  Port=5
  In6 : Inport  Port=6
  In7 : Inport  Port=7
  In8 : Inport  Port=8
  In9 : Inport  Port=9
  In10 : Inport  Port=10
  In11 : Inport  Port=11
  In12 : Inport  Port=12
  In13 : Inport  Port=13
  In14 : Inport  Port=14
  In15 : Inport  Port=15
  In17 : Inport  Port=16
  In19 : Inport  Port=17
  In16 : Inport  Port=18
  In18 : Inport  Port=19
  In20 : Inport  Port=20
  In21 : Inport  Port=21
  In22 : Inport  Port=22
  In23 : Inport  Port=23
  In24 : Inport  Port=24
  In25 : Inport  Port=25
  In26 : Inport  Port=26
  In27 : Inport  Port=27
  In28 : Inport  Port=28
  In29 : Inport  Port=29
  In30 : Inport  Port=30
  In31 : Inport  Port=31
  In32 : Inport  Port=32
  Add{,2,4,6,8,10,12,14,16,18,20,22,24,26,28,30} (16 alike) : Sum  OutDataTypeStr=fixed  RndMeth=Round
  Add{1,3,5,7,9,11,13,15,17,19,21,23,25,27,29,31} (16 alike) : Sum  Inputs=+-  OutDataTypeStr=fixed  RndMeth=Round
  Constant1 : Constant  Value=exp(-1j*pi/8)  OutDataTypeStr=fixed  SampleTime=-1
  Constant10 : Constant  Value=exp(-1j*pi*13/16)  OutDataTypeStr=fixed  SampleTime=-1
  Constant12 : Constant  Value=exp(-1j*7*pi/8)  OutDataTypeStr=fixed  SampleTime=-1
  Constant13 : Constant  Value=exp(-1j*pi*15/16)  OutDataTypeStr=fixed  SampleTime=-1
  Constant2 : Constant  Value=exp(-1j*pi/16)  OutDataTypeStr=fixed  SampleTime=-1
  Constant3 : Constant  Value=exp(-1j*pi*3/16)  OutDataTypeStr=fixed  SampleTime=-1
  Constant4 : Constant  Value=exp(-1j*pi*5/16)  OutDataTypeStr=fixed  SampleTime=-1
  Constant5 : Constant  Value=exp(-1j*pi*3/8)  OutDataTypeStr=fixed  SampleTime=-1
  Constant6 : Constant  Value=exp(-1j*pi*5/8)  OutDataTypeStr=fixed  SampleTime=-1
  Constant7 : Constant  Value=exp(-1j*pi*7/16)  OutDataTypeStr=fixed  SampleTime=-1
  Constant8 : Constant  Value=exp(-1j*pi*9/16)  OutDataTypeStr=fixed  SampleTime=-1
  Constant9 : Constant  Value=exp(-1j*pi*11/16)  OutDataTypeStr=fixed  SampleTime=-1
  Delay{,9..15,17,20..21,25,28..47,49,51} (34 alike) : Delay  DelayLength=1
  Delay{1..8,16,18..19,22..24,26..27,48,50} (18 alike) : Delay  DelayLength=3
  FFT16 : Subsystem
  FFT16_1 : Subsystem
  complexmult : Subsystem
  complexmult1 : Subsystem
  complexmult10 : Subsystem
  complexmult11 : Subsystem
  complexmult2 : Subsystem
  complexmult3 : Subsystem
  complexmult4 : Subsystem
  complexmult5 : Subsystem
  complexmult6 : Subsystem
  complexmult7 : Subsystem
  complexmult8 : Subsystem
  complexmult9 : Subsystem
  multByExp(-j*Pi/4) : Subsystem
  multByExp(-j*Pi/4)1 : Subsystem
  multByMinusJ : Subsystem
  multByMinusJ3 : Subsystem
  x0 : Outport  VectorParamsAs1DForOutWhenUnconnected=off
  x1 : Outport  Port=2  VectorParamsAs1DForOutWhenUnconnected=off
  x2 : Outport  Port=3  VectorParamsAs1DForOutWhenUnconnected=off
  x3 : Outport  Port=4  VectorParamsAs1DForOutWhenUnconnected=off
  x4 : Outport  Port=5  VectorParamsAs1DForOutWhenUnconnected=off
  x5 : Outport  Port=6  VectorParamsAs1DForOutWhenUnconnected=off
  x6 : Outport  Port=7  VectorParamsAs1DForOutWhenUnconnected=off
  x7 : Outport  Port=8  VectorParamsAs1DForOutWhenUnconnected=off
  x8 : Outport  Port=9  VectorParamsAs1DForOutWhenUnconnected=off
  x9 : Outport  Port=10  VectorParamsAs1DForOutWhenUnconnected=off
  x10 : Outport  Port=11  VectorParamsAs1DForOutWhenUnconnected=off
  x11 : Outport  Port=12  VectorParamsAs1DForOutWhenUnconnected=off
  x12 : Outport  Port=13  VectorParamsAs1DForOutWhenUnconnected=off
  x13 : Outport  Port=14  VectorParamsAs1DForOutWhenUnconnected=off
  x14 : Outport  Port=15  VectorParamsAs1DForOutWhenUnconnected=off
  x15 : Outport  Port=16  VectorParamsAs1DForOutWhenUnconnected=off
  x16 : Outport  Port=17  VectorParamsAs1DForOutWhenUnconnected=off
  x17 : Outport  Port=18  VectorParamsAs1DForOutWhenUnconnected=off
  x18 : Outport  Port=19  VectorParamsAs1DForOutWhenUnconnected=off
  x19 : Outport  Port=20  VectorParamsAs1DForOutWhenUnconnected=off
  x20 : Outport  Port=21  VectorParamsAs1DForOutWhenUnconnected=off
  x21 : Outport  Port=22  VectorParamsAs1DForOutWhenUnconnected=off
  x22 : Outport  Port=23  VectorParamsAs1DForOutWhenUnconnected=off
  x23 : Outport  Port=24  VectorParamsAs1DForOutWhenUnconnected=off
  x24 : Outport  Port=25  VectorParamsAs1DForOutWhenUnconnected=off
  x25 : Outport  Port=26  VectorParamsAs1DForOutWhenUnconnected=off
  x26 : Outport  Port=27  VectorParamsAs1DForOutWhenUnconnected=off
  x27 : Outport  Port=28  VectorParamsAs1DForOutWhenUnconnected=off
  x28 : Outport  Port=29  VectorParamsAs1DForOutWhenUnconnected=off
  x29 : Outport  Port=30  VectorParamsAs1DForOutWhenUnconnected=off
  x30 : Outport  Port=31  VectorParamsAs1DForOutWhenUnconnected=off
  x31 : Outport  Port=32  VectorParamsAs1DForOutWhenUnconnected=off
  wires:
  Delay37/1 -> x30/1
  Delay34/1 -> x29/1
  Delay33/1 -> x28/1
  Delay46/1 -> x27/1
  Delay45/1 -> x26/1
  Delay44/1 -> x25/1
  Delay43/1 -> x24/1
  Delay15/1 -> x23/1
  Delay14/1 -> x22/1
  Delay11/1 -> x21/1
  Delay10/1 -> x20/1
  Delay31/1 -> x19/1
  Delay38/1 -> x31/1
  Delay25/1 -> x5/1
  Delay21/1 -> x4/1
  Delay30/1 -> x18/1
  Delay29/1 -> x17/1
  Delay28/1 -> x16/1
  Delay36/1 -> x15/1
  Delay35/1 -> x14/1
  Delay42/1 -> x13/1
  Delay41/1 -> x12/1
  Delay40/1 -> x11/1
  Delay39/1 -> x10/1
  Delay47/1 -> x9/1
  Delay12/1 -> x6/1
  Delay32/1 -> x8/1
  Delay13/1 -> x7/1
  Delay20/1 -> x3/1
  Delay17/1 -> x2/1
  Delay9/1 -> x1/1
  Delay/1 -> x0/1
  complexmult11/1(Out1) -> Add23/2, Add22/2
  complexmult10/1(Out1) -> Add20/2, Add21/2
  complexmult9/1(Out1) -> Add19/2, Add18/2
  Delay51/1 -> Add31/2, Add30/2
  complexmult8/1(Out1) -> Add29/2, Add28/2
  complexmult7/1(Out1) -> Add26/2, Add27/2
  complexmult6/1(Out1) -> Add24/2, Add25/2
  Delay50/1 -> Add17/2, Add16/2
  complexmult5/1(Out1) -> Add15/2, Add14/2
  complexmult4/1(Out1) -> Add13/2, Add12/2
  complexmult3/1(Out1) -> Add10/2, Add11/2
  Constant13/1 -> complexmult11/2(In3)
  Constant12/1 -> complexmult10/2(In3)
  FFT16_1/16(x15) -> complexmult11/1(x1)
  FFT16_1/15(x14) -> complexmult10/1(x1)
  FFT16_1/13(x12) -> multByExp(-j*Pi/4)1/1(x4)
  FFT16_1/14(x13) -> complexmult9/1(x1)
  Constant10/1 -> complexmult9/2(In3)
  Constant9/1 -> complexmult8/2(In3)
  FFT16_1/12(x11) -> complexmult8/1(x1)
  Constant6/1 -> complexmult7/2(In3)
  FFT16_1/11(x10) -> complexmult7/1(x1)
  Constant8/1 -> complexmult6/2(In3)
  FFT16_1/10(x9) -> complexmult6/1(x1)
  Constant7/1 -> complexmult5/2(In3)
  FFT16_1/8(x7) -> complexmult5/1(x1)
  Constant5/1 -> complexmult4/2(In3)
  FFT16_1/7(x6) -> complexmult4/1(x1)
  Constant4/1 -> complexmult3/2(In3)
  FFT16_1/6(x5) -> complexmult3/1(x1)
  multByMinusJ3/1(Out1) -> Delay51/1
  multByExp(-j*Pi/4)1/1(Out1) -> multByMinusJ3/1(In1)
  FFT16_1/9(x8) -> multByMinusJ/1(x4)
  multByMinusJ/1(Out1) -> Delay50/1
  Delay49/1 -> Add8/2, Add9/2
  FFT16_1/5(x4) -> multByExp(-j*Pi/4)/1(x4)
  multByExp(-j*Pi/4)/1(Out1) -> Delay49/1
  complexmult2/1(Out1) -> Add6/2, Add7/2
  Constant3/1 -> complexmult2/2(In3)
  FFT16_1/4(x3) -> complexmult2/1(x1)
  complexmult1/1(Out1) -> Add4/2, Add5/2
  Constant1/1 -> complexmult1/2(In3)
  FFT16_1/3(x2) -> complexmult1/1(x1)
  complexmult/1(Out1) -> Add2/2, Add3/2
  Constant2/1 -> complexmult/2(In3)
  FFT16_1/2(x1) -> complexmult/1(x1)
  Delay8/1 -> Add23/1, Add22/1
  Delay7/1 -> Add20/1, Add21/1
  Delay6/1 -> Add19/1, Add18/1
  Delay5/1 -> Add30/1, Add31/1
  Delay1/1 -> Add29/1, Add28/1
  Delay3/1 -> Add27/1, Add26/1
  Delay2/1 -> Add25/1, Add24/1
  Delay4/1 -> Add17/1, Add16/1
  Delay27/1 -> Add14/1, Add15/1
  Delay26/1 -> Add13/1, Add12/1
  Delay24/1 -> Add10/1, Add11/1
  Delay23/1 -> Add9/1, Add8/1
  Delay16/1 -> Add6/1, Add7/1
  Delay19/1 -> Add4/1, Add5/1
  Delay18/1 -> Add2/1, Add3/1
  Delay48/1 -> Add1/2, Add/2
  FFT16_1/1(x0) -> Delay48/1
  Delay22/1 -> Add1/1, Add/1
  Add27/1 -> Delay45/1
  Add16/1 -> Delay32/1
  Add23/1 -> Delay38/1
  Add30/1 -> Delay41/1
  Add24/1 -> Delay47/1
  Add28/1 -> Delay40/1
  Add22/1 -> Delay36/1
  Add26/1 -> Delay39/1
  Add31/1 -> Delay33/1
  Add17/1 -> Delay43/1
  Add29/1 -> Delay46/1
  Add19/1 -> Delay34/1
  Add25/1 -> Delay44/1
  Add21/1 -> Delay37/1
  Add20/1 -> Delay35/1
  Add18/1 -> Delay42/1
  Add2/1 -> Delay9/1
  Add9/1 -> Delay10/1
  Add8/1 -> Delay21/1
  Add14/1 -> Delay13/1
  Add12/1 -> Delay12/1
  Add15/1 -> Delay15/1
  Add3/1 -> Delay29/1
  Add4/1 -> Delay17/1
  Add10/1 -> Delay25/1
  Add/1 -> Delay/1
  Add5/1 -> Delay30/1
  Add13/1 -> Delay14/1
  Add6/1 -> Delay20/1
  Add11/1 -> Delay11/1
  Add7/1 -> Delay31/1
  Add1/1 -> Delay28/1
  FFT16/16(x15) -> Delay8/1
  FFT16/9(x8) -> Delay4/1
  FFT16/15(x14) -> Delay7/1
  FFT16/10(x9) -> Delay2/1
  FFT16/14(x13) -> Delay6/1
  FFT16/11(x10) -> Delay3/1
  FFT16/13(x12) -> Delay5/1
  FFT16/12(x11) -> Delay1/1
  FFT16/8(x7) -> Delay27/1
  FFT16/7(x6) -> Delay26/1
  FFT16/6(x5) -> Delay24/1
  FFT16/5(x4) -> Delay23/1
  FFT16/4(x3) -> Delay16/1
  FFT16/3(x2) -> Delay19/1
  FFT16/2(x1) -> Delay18/1
  FFT16/1(x0) -> Delay22/1
  In32/1 -> FFT16_1/16(In16)
  In30/1 -> FFT16_1/15(In15)
  In28/1 -> FFT16_1/14(In14)
  In26/1 -> FFT16_1/13(In13)
  In24/1 -> FFT16_1/12(In12)
  In22/1 -> FFT16_1/11(In11)
  In20/1 -> FFT16_1/10(In10)
  In16/1 -> FFT16_1/9(In9)
  In17/1 -> FFT16_1/8(In8)
  In14/1 -> FFT16_1/7(In7)
  In12/1 -> FFT16_1/6(In6)
  In10/1 -> FFT16_1/5(In5)
  In8/1 -> FFT16_1/4(In4)
  In6/1 -> FFT16_1/3(In3)
  In4/1 -> FFT16_1/2(In2)
  In2/1 -> FFT16_1/1(In1)
  In31/1 -> FFT16/16(In16)
  In29/1 -> FFT16/15(In15)
  In27/1 -> FFT16/14(In14)
  In25/1 -> FFT16/13(In13)
  In23/1 -> FFT16/12(In12)
  In21/1 -> FFT16/11(In11)
  In18/1 -> FFT16/10(In10)
  In19/1 -> FFT16/9(In9)
  In15/1 -> FFT16/8(In8)
  In13/1 -> FFT16/7(In7)
  In11/1 -> FFT16/6(In6)
  In9/1 -> FFT16/5(In5)
  In7/1 -> FFT16/4(In4)
  In5/1 -> FFT16/3(In3)
  In3/1 -> FFT16/2(In2)
  In1/1 -> FFT16/1(In1)
